simulink model "cruise_ground_up_final"  (R2021a)
settings: Solver=VariableStepAuto  StartTime=0  StopTime=10.0  RelTol=1e-3
model workspace (MAT data in the model file):
  aeroCoeff.Cl0 = 0
  aeroCoeff.Cl_beta = -0.036269164
  aeroCoeff.Cl_da = -0.1109919434
  aeroCoeff.Cl_dr = 0.1739783018
  aeroCoeff.Cl_p = -0.7949096926
  aeroCoeff.Cl_r = 0.2014971632
  aeroCoeff.Cm0 = 0
  aeroCoeff.Cm_alpha = -0.43
  aeroCoeff.Cm_de = -1.553
  aeroCoeff.Cm_q = -7.04
  aeroCoeff.Cn0 = 0
  aeroCoeff.Cn_beta = 0.048869199
  aeroCoeff.Cn_da = 0.0182026787
  aeroCoeff.Cn_dr = -0.3910440741
  aeroCoeff.Cn_p = -0.0359727396
  aeroCoeff.Cn_r = -0.0735610276
  aeroCoeff.Cx0 = 0
  aeroCoeff.Cx_alpha = 0.4653
  aeroCoeff.Cx_q = 0
  aeroCoeff.Cx_de = 0
  aeroCoeff.Cy0 = 0
  aeroCoeff.Cy_beta = -0.1609874369
  aeroCoeff.Cy_da = 0
  aeroCoeff.Cy_dr = 0.9151416544
  aeroCoeff.Cy_p = -0.0237997869
  aeroCoeff.Cy_r = 0.1375812867
  aeroCoeff.Cz0 = -1.136
  aeroCoeff.Cz_alpha = -5.16
  aeroCoeff.Cz_de = -0.6238
  aeroCoeff.Cz_q = -3.86
  aeroCoeff.Cx_u = -0.2199
  aeroCoeff.Cz_u = -2.272
  aeroCoeff.Cm_u = 0
  aeroCoeff.Cx_adot = 0
  aeroCoeff.Cz_adot = 1.43
  aeroCoeff.Cm_adot = -3.7
  aeroCoeff.V0 = 59.9
  environment.EarthRefAlt = 0
  initCond.x0 = [0 0 -1000]
  initCond.v0 = [59.9 0 0]
  initCond.euler0 = [0 0 0]
  initCond.w0 = [0 0 0]
  inputs0.time = 0
  inputs0.signals(1).dimensions = 1
  inputs0.signals(1).values = -0.104711430294
  inputs0.signals(2).dimensions = 1
  inputs0.signals(2).values = -0.0698725229544
  inputs0.signals(3).dimensions = 1
  inputs0.signals(3).values = -0.000215042330254
  states0.time = 0
  states0.signals(1).values = [0 0 -1000]
  states0.signals(1).dimensions = 3
  states0.signals(1).label = 'CSTATE'
  states0.signals(1).blockName = 'asb6DOFAirframeTemplate/6DOF EOM/6DOF (Euler Angles)/xe,ye,ze'
  states0.signals(1).stateName = ''
  states0.signals(1).inReferencedModel = 0
  states0.signals(1).sampleTime = [0 0]
  states0.signals(2).values = [0.128665353089 0.259337659946 -0.178947917154]
  states0.signals(2).dimensions = 3
  states0.signals(2).label = 'CSTATE'
  states0.signals(2).blockName = 'asb6DOFAirframeTemplate/6DOF EOM/6DOF (Euler Angles)/Calculate DCM &
    | Euler Angles/phi
    | theta
    | psi'
  states0.signals(2).stateName = ''
  states0.signals(2).inReferencedModel = 0
  states0.signals(2).sampleTime = [0 0]
  states0.signals(3).values = [36.9119692666 8.10720863264 8.82591882596]
  states0.signals(3).dimensions = 3
  states0.signals(3).label = 'CSTATE'
  states0.signals(3).blockName = 'asb6DOFAirframeTemplate/6DOF EOM/6DOF (Euler Angles)/ub,vb,wb'
  states0.signals(3).stateName = ''
  states0.signals(3).inReferencedModel = 0
  states0.signals(3).sampleTime = [0 0]
  states0.signals(4).values = [0 0 0]
  states0.signals(4).dimensions = 3
  states0.signals(4).label = 'CSTATE'
  states0.signals(4).blockName = 'asb6DOFAirframeTemplate/6DOF EOM/6DOF (Euler Angles)/p,q,r '
  states0.signals(4).stateName = ''
  states0.signals(4).inReferencedModel = 0
  states0.signals(4).sampleTime = [0 0]
  states0.signals(5).values = [0 0]
  states0.signals(5).dimensions = 2
  states0.signals(5).label = 'CSTATE'
  states0.signals(5).blockName = 'asb6DOFAirframeTemplate/Environment Model/Dryden Wind Turbulence Model 
    | (Continuous (+q +r))/Filters on velocities/Hwgw(s)/wg_p1'
  states0.signals(5).stateName = ''
  states0.signals(5).inReferencedModel = 0
  states0.signals(5).sampleTime = [0 0]
  states0.signals(6).values = [0 0]
  states0.signals(6).dimensions = 2
  states0.signals(6).label = 'CSTATE'
  states0.signals(6).blockName = 'asb6DOFAirframeTemplate/Environment Model/Dryden Wind Turbulence Model 
    | (Continuous (+q +r))/Filters on velocities/Hwgw(s)/wg_p2'
  states0.signals(6).stateName = ''
  states0.signals(6).inReferencedModel = 0
  states0.signals(6).sampleTime = [0 0]
  states0.signals(7).values = [0 0]
  states0.signals(7).dimensions = 2
  states0.signals(7).label = 'CSTATE'
  states0.signals(7).blockName = 'asb6DOFAirframeTemplate/Environment Model/Dryden Wind Turbulence Model 
    | (Continuous (+q +r))/Filters on velocities/Hvgw(s)/vg_p1'
  states0.signals(7).stateName = ''
  states0.signals(7).inReferencedModel = 0
  states0.signals(7).sampleTime = [0 0]
  states0.signals(8).values = [0 0]
  states0.signals(8).dimensions = 2
  states0.signals(8).label = 'CSTATE'
  states0.signals(8).blockName = 'asb6DOFAirframeTemplate/Environment Model/Dryden Wind Turbulence Model 
    | (Continuous (+q +r))/Filters on velocities/Hvgw(s)/vgw_p2'
  states0.signals(8).stateName = ''
  states0.signals(8).inReferencedModel = 0
  states0.signals(8).sampleTime = [0 0]
  states0.signals(9).values = [0 0]
  states0.signals(9).dimensions = 2
  states0.signals(9).label = 'CSTATE'
  states0.signals(9).blockName = 'asb6DOFAirframeTemplate/Environment Model/Dryden Wind Turbulence Model 
    | (Continuous (+q +r))/Filters on velocities/Hugw(s)/ug_p'
  states0.signals(9).stateName = ''
  states0.signals(9).inReferencedModel = 0
  states0.signals(9).sampleTime = [0 0]
  states0.signals(10).values = [0 0]
  states0.signals(10).dimensions = 2
  states0.signals(10).label = 'CSTATE'
  states0.signals(10).blockName = 'asb6DOFAirframeTemplate/Environment Model/Dryden Wind Turbulence Model 
    | (Continuous (+q +r))/Filters on angular rates/Hrgw/rgw_p'
  states0.signals(10).stateName = ''
  states0.signals(10).inReferencedModel = 0
  states0.signals(10).sampleTime = [0 0]
  states0.signals(11).values = [0 0]
  states0.signals(11).dimensions = 2
  states0.signals(11).label = 'CSTATE'
  states0.signals(11).blockName = 'asb6DOFAirframeTemplate/Environment Model/Dryden Wind Turbulence Model 
    | (Continuous (+q +r))/Filters on angular rates/Hqgw/qgw_p'
  states0.signals(11).stateName = ''
  states0.signals(11).inReferencedModel = 0
  states0.signals(11).sampleTime = [0 0]
  states0.signals(12).values = [0 0]
  states0.signals(12).dimensions = 2
  states0.signals(12).label = 'CSTATE'
  states0.signals(12).blockName = 'asb6DOFAirframeTemplate/Environment Model/Dryden Wind Turbulence Model 
    | (Continuous (+q +r))/Filters on angular rates/Hpgw/pgw_p'
  states0.signals(12).stateName = ''
  states0.signals(12).inReferencedModel = 0
  states0.signals(12).sampleTime = [0 0]
  vehicle.Sref = 24.2
  vehicle.cbar = 2.022
  vehicle.bref = 8.7036787674
  vehicle.CG = [0 0 0]
  vehicle.CP = [0 0 0]
  vehicle.inertia = [11509.7158987  0  121.163701749; 0  18221.7353845  0; -121.163701749  0  28644.1528969]
  vehicle.acMass = 4547.8
  vehicle.Thrust = 2300
  vehicle.aileron_max = 0.523598775598
  vehicle.aileron_min = -0.523598775598
  vehicle.elevator_max = 0.305432619099
  vehicle.elevator_min = -0.305432619099
  vehicle.rudder_max = 0.436332312999
  vehicle.rudder_min = -0.436332312999
values from neighbouring files (symbols this model uses):
  aeroCoeff = struct    [cruise_from_template_variables.m]    (also in cruise_ground_up_variables.m; cruise_ground_up_variables_cessna.m)
  vehicle = struct    [cruise_from_template_variables.m]    (also in cruise_ground_up_variables.m; cruise_ground_up_variables_cessna.m)
libraries: aerolibasang x2, pid_lib x2, aerolibadyn x1, aerolibatmos2 x1, shared6dof x1
settings Model: OrderedModelArguments=off  Creator=jakob  LastModifiedBy=jakob
settings DataIOCC: SaveFormat=StructureWithTime
settings OptimizationCC: BlockReduction=off  BufferReuse=off
settings DebuggingCC: AlgebraicLoopMsg=none  UnconnectedInputMsg=none  UnconnectedOutputMsg=none  UnconnectedLineMsg=none

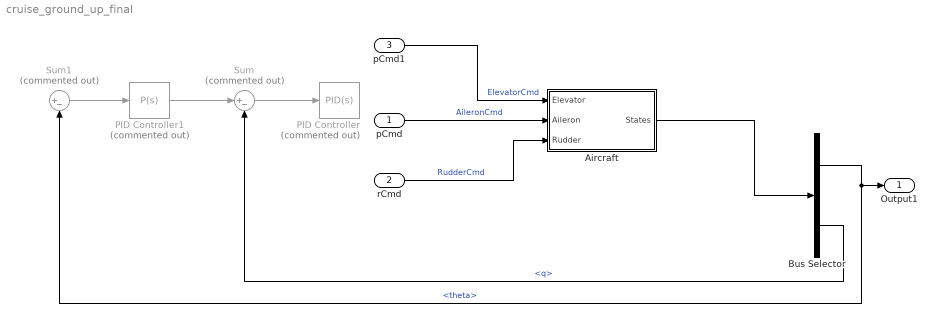
== system cruise_ground_up_final ==
  pCmd : Inport
  rCmd : Inport  Port=2
  pCmd1 : Inport  Port=3
  Aircraft : Subsystem
  Bus Selector : BusSelector  OutputSignals=phi,theta,psi,p,q,r
  PID Controller : pid_lib/PID Controller  Commented=on  Controller=PID  Form=Parallel  TimeDomain=Continuous-time  UseExternalTs=off  SampleTime=-1  IntegratorMethod=Forward Euler  FilterMethod=Forward Euler  ControllerParametersSource=internal  P=5.93921681747146  I=63.1505692304765  D=-0.00231186106807805  UseFilter=on  N=2569.01978214849  TunerSelectOption=Transfer Function Based (PID Tuner App)  InitialConditionSource=internal  InitialConditionForIntegrator=0  InitialConditionForFilter=0  DifferentiatorICPrevScaledInput=0  ExternalReset=none  TrackingMode=off  Kt=1  LimitOutput=off  SatLimitsSource=internal  UpperSaturationLimit=inf  LowerSaturationLimit=-inf  LinearizeAsGain=on  AntiWindupMode=none  Kb=1  POutMin=[]  POutMax=[]  IOutMin=[]  IOutMax=[]  DOutMin=[]  DOutMax=[]  NOutMin=[]  NOutMax=[]  SumOutMin=[]  SumOutMax=[]  SaturationOutMin=[]  SaturationOutMax=[]  PParamMin=[]  PParamMax=[]  IParamMin=[]  IParamMax=[]  DParamMin=[]  DParamMax=[]  NParamMin=[]  NParamMax=[]  KbParamMin=[]  KbParamMax=[]  KtParamMin=[]  KtParamMax=[]  KbOutMin=[]  KbOutMax=[]  KtOutMin=[]  KtOutMax=[]  IntegratorOutMin=[]  IntegratorOutMax=[]  FilterOutMin=[]  FilterOutMax=[]  SumI1OutMin=[]  SumI1OutMax=[]  SumI2OutMin=[]  SumI2OutMax=[]  SumI3OutMin=[]  SumI3OutMax=[]  SumI4OutMin=[]  SumI4OutMax=[]  SumDOutMin=[]  SumDOutMax=[]  DifferentiatorOutMin=[]  DifferentiatorOutMax=[]  FilterDiffOutCoefMin=[]  FilterDiffOutCoefMax=[]  ReciprocalOutMin=[]  ReciprocalOutMax=[]  SumDenOutMin=[]  SumDenOutMax=[]  SumNumOutMin=[]  SumNumOutMax=[]  DivideOutMin=[]  DivideOutMax=[]  UdiffTsProdOutMin=[]  UdiffTsProdOutMax=[]  NTsProdOutMin=[]  NTsProdOutMax=[]  UintegralTsProdOutMin=[]  UintegralTsProdOutMax=[]  UngainTsProdOutMin=[]  UngainTsProdOutMax=[]  IntegratorContinuousStateAttributes=''  IntegratorStateMustResolveToSignalObject=off  IntegratorRTWStateStorageClass=Auto  FilterContinuousStateAttributes=''  FilterStateMustResolveToSignalObject=off  FilterRTWStateStorageClass=Auto  ParallelPVariant=InternalParameters  IdealPVariant=Disabled  IVariant=InternalParameters  DVariant=InternalParameters  IntegratorVariant=Continuous  SatVariant=Disabled  AWVariant=Passthrough  PCopyVariant=Disabled  TRVariant=Disabled  FdbkBlocksVariant=Forward  IdealPFdbkVariant=Disabled  SatFdbkVariant=Disabled  DerivativeFilterVariant=ContFilter  NVariant=InternalParameters  NCopyVariant=Disabled  FilterICVariant=InternalICsFilter  IntegratorICVariant=InternalICs  ExternalResetVariant=Disabled  TRSumVariant=Passthrough  SumFdbkVariant=Disabled  SumVariant=Sum_PID  TsampFilterVariant=InternalTs  TsampNgainVariant=Passthrough  TsampIntegralVariant=Passthrough  ExternalSaturationOutDataTypeStr=Inherit: Same as second input
  PID Controller1 : pid_lib/PID Controller  Commented=on  Controller=P  Form=Parallel  TimeDomain=Continuous-time  UseExternalTs=off  SampleTime=-1  IntegratorMethod=Forward Euler  FilterMethod=Forward Euler  ControllerParametersSource=internal  P=3.47272160532588  I=1  D=0  UseFilter=on  N=100  TunerSelectOption=Transfer Function Based (PID Tuner App)  InitialConditionSource=internal  InitialConditionForIntegrator=0  InitialConditionForFilter=0  DifferentiatorICPrevScaledInput=0  ExternalReset=none  TrackingMode=off  Kt=1  LimitOutput=off  SatLimitsSource=internal  UpperSaturationLimit=inf  LowerSaturationLimit=-inf  LinearizeAsGain=on  AntiWindupMode=none  Kb=1  POutMin=[]  POutMax=[]  IOutMin=[]  IOutMax=[]  DOutMin=[]  DOutMax=[]  NOutMin=[]  NOutMax=[]  SumOutMin=[]  SumOutMax=[]  SaturationOutMin=[]  SaturationOutMax=[]  PParamMin=[]  PParamMax=[]  IParamMin=[]  IParamMax=[]  DParamMin=[]  DParamMax=[]  NParamMin=[]  NParamMax=[]  KbParamMin=[]  KbParamMax=[]  KtParamMin=[]  KtParamMax=[]  KbOutMin=[]  KbOutMax=[]  KtOutMin=[]  KtOutMax=[]  IntegratorOutMin=[]  IntegratorOutMax=[]  FilterOutMin=[]  FilterOutMax=[]  SumI1OutMin=[]  SumI1OutMax=[]  SumI2OutMin=[]  SumI2OutMax=[]  SumI3OutMin=[]  SumI3OutMax=[]  SumI4OutMin=[]  SumI4OutMax=[]  SumDOutMin=[]  SumDOutMax=[]  DifferentiatorOutMin=[]  DifferentiatorOutMax=[]  FilterDiffOutCoefMin=[]  FilterDiffOutCoefMax=[]  ReciprocalOutMin=[]  ReciprocalOutMax=[]  SumDenOutMin=[]  SumDenOutMax=[]  SumNumOutMin=[]  SumNumOutMax=[]  DivideOutMin=[]  DivideOutMax=[]  UdiffTsProdOutMin=[]  UdiffTsProdOutMax=[]  NTsProdOutMin=[]  NTsProdOutMax=[]  UintegralTsProdOutMin=[]  UintegralTsProdOutMax=[]  UngainTsProdOutMin=[]  UngainTsProdOutMax=[]  IntegratorContinuousStateAttributes=''  IntegratorStateMustResolveToSignalObject=off  IntegratorRTWStateStorageClass=Auto  FilterContinuousStateAttributes=''  FilterStateMustResolveToSignalObject=off  FilterRTWStateStorageClass=Auto  ParallelPVariant=InternalParameters  IdealPVariant=Disabled  IVariant=Disabled  DVariant=Disabled  IntegratorVariant=Disabled  SatVariant=Disabled  AWVariant=Disabled  PCopyVariant=Disabled  TRVariant=Disabled  FdbkBlocksVariant=Forward  IdealPFdbkVariant=Disabled  SatFdbkVariant=Disabled  DerivativeFilterVariant=Disabled  NVariant=Disabled  NCopyVariant=Disabled_SignalSpec  FilterICVariant=Disabled  IntegratorICVariant=Disabled  ExternalResetVariant=Disabled  TRSumVariant=Passthrough  SumFdbkVariant=Disabled  SumVariant=Passthrough_P  TsampFilterVariant=InternalTs  TsampNgainVariant=Passthrough  TsampIntegralVariant=Disabled_SignalSpec  ExternalSaturationOutDataTypeStr=Inherit: Same as second input
  Sum : Sum  Commented=on  Inputs=|+-
  Sum1 : Sum  Commented=on  Inputs=|+-
  Output1 : Outport
  wires:
  Aircraft/1(States) -> Bus Selector/1
  pCmd/1 -> Aircraft/2(Aileron)  "AileronCmd"
  rCmd/1 -> Aircraft/3(Rudder)  "RudderCmd"
  Sum/1 -> PID Controller/1
  Bus Selector/5 -> Sum/2  "<q>"
  Sum1/1 -> PID Controller1/1
  PID Controller1/1 -> Sum/1
  Bus Selector/2 -> Output1/1, Sum1/2  "<theta>"
  pCmd1/1 -> Aircraft/1(Elevator)  "ElevatorCmd"

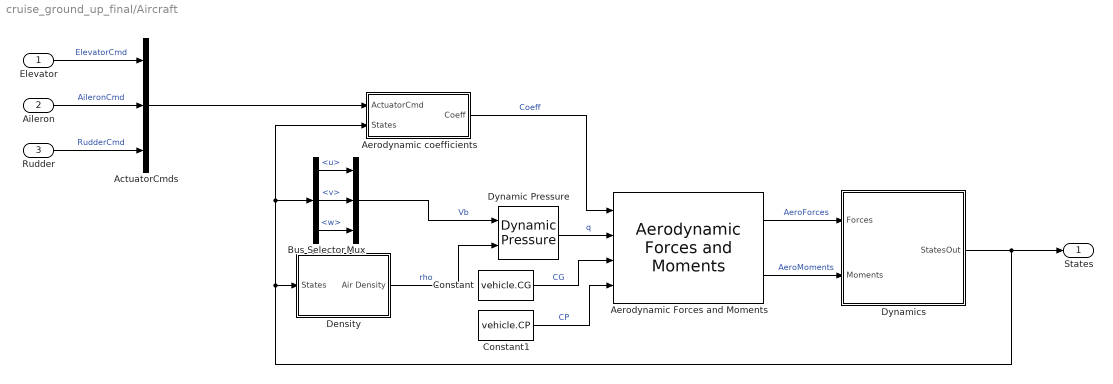
== system cruise_ground_up_final/Aircraft ==
  Elevator : Inport
  Aileron : Inport  Port=2
  Rudder : Inport  Port=3
  ActuatorCmds : BusCreator  Inputs=3
  "Aerodynamic Forces and Moments " : aerolibadyn/Aerodynamic Forces and Moments   inputAxes=Body  outputForceAxes=Body  outputMomentAxes=Body  S=vehicle.Sref  b=vehicle.bref  cbar=vehicle.cbar
  Aerodynamic coefficients : Subsystem
  Bus Selector : BusSelector  OutputSignals=u,v,w
  Constant : Constant  Value=vehicle.CG
  Constant1 : Constant  Value=vehicle.CP
  Density : Subsystem
  Dynamic Pressure : aerolibasang/Dynamic Pressure
  Dynamics : Subsystem
  Mux : Mux  Inputs=3
  States : Outport
  wires:
  "Aerodynamic Forces and Moments "/1 -> Dynamics/1(Forces)  "AeroForces"
  Aileron/1 -> ActuatorCmds/2  "AileronCmd"
  ActuatorCmds/1 -> Aerodynamic coefficients/1(ActuatorCmd)
  Rudder/1 -> ActuatorCmds/3  "RudderCmd"
  Dynamic Pressure/1 -> "Aerodynamic Forces and Moments "/2  "q"
  Elevator/1 -> ActuatorCmds/1  "ElevatorCmd"
  Aerodynamic coefficients/1(Coeff) -> "Aerodynamic Forces and Moments "/1  "Coeff"
  Dynamics/1(StatesOut) -> States/1, Aerodynamic coefficients/2(States), Bus Selector/1, Density/1(States)
  "Aerodynamic Forces and Moments "/2 -> Dynamics/2(Moments)  "AeroMoments"
  Density/1(Air Density) -> Dynamic Pressure/2  "rho"
  Constant/1 -> "Aerodynamic Forces and Moments "/3  "CG"
  Mux/1 -> Dynamic Pressure/1  "Vb"
  Constant1/1 -> "Aerodynamic Forces and Moments "/4  "CP"
  Bus Selector/2 -> Mux/2  "<v>"
  Bus Selector/1 -> Mux/1  "<u>"
  Bus Selector/3 -> Mux/3  "<w>"

== system cruise_ground_up_final/Aircraft/Aerodynamic coefficients ==
  ActuatorCmd : Inport
  States : Inport  Port=2
  Control derivatives : Subsystem
  Stability derivatives : Subsystem
  Sum : Sum  Inputs=|++
  Coeff : Outport
  wires:
  Sum/1 -> Coeff/1
  Stability derivatives/1(Coeff) -> Sum/2
  Control derivatives/1(Coeff) -> Sum/1
  States/1 -> Stability derivatives/1(StatesOut)
  ActuatorCmd/1 -> Control derivatives/1(ActuatorCmd)

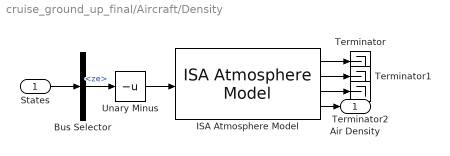
== system cruise_ground_up_final/Aircraft/Density ==
  States : Inport
  Bus Selector : BusSelector  OutputSignals=ze
  ISA Atmosphere Model : aerolibatmos2/ISA Atmosphere Model  custom=off  g=9.80665  gamma=1.4  R=287.0531  L=0.0065  h_trop=11000  h_strat=20000  rho0=1.225  P0=101325  T0=288.15  h0=0
  Terminator : Terminator
  Terminator1 : Terminator
  Terminator2 : Terminator
  Unary Minus : UnaryMinus
  Air Density : Outport
  wires:
  ISA Atmosphere Model/3 -> Terminator2/1
  ISA Atmosphere Model/2 -> Terminator1/1
  ISA Atmosphere Model/4 -> Air Density/1
  Bus Selector/1 -> Unary Minus/1  "<ze>"
  Unary Minus/1 -> ISA Atmosphere Model/1
  ISA Atmosphere Model/1 -> Terminator/1
  States/1 -> Bus Selector/1

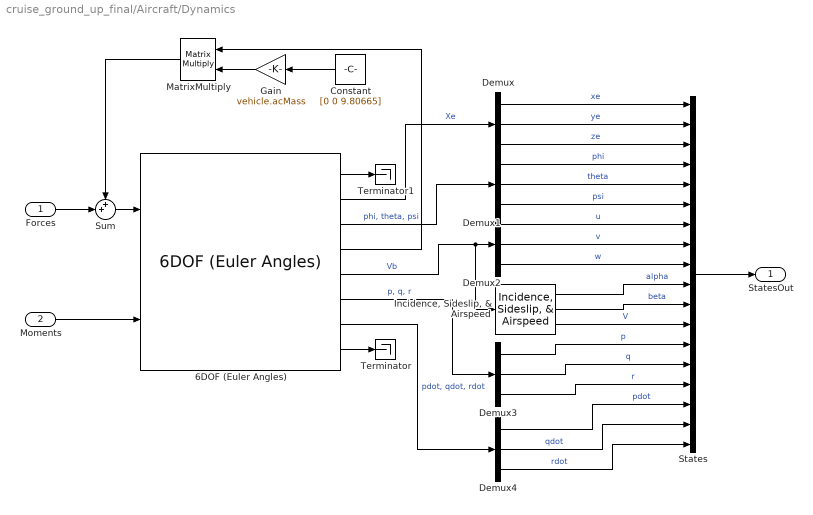
== system cruise_ground_up_final/Aircraft/Dynamics ==
  Forces : Inport
  Moments : Inport  Port=2
  6DOF (Euler Angles) : shared6dof/6DOF (Euler Angles)  units=Metric (MKS)  mtype=Fixed  rep=Euler Angles  xme_0=initCond.x0  Vm_0=initCond.v0  eul_0=initCond.euler0  pm_0=initCond.w0  mass_0=vehicle.acMass  mass_e=0.5  mass_f=2.0  inertia=vehicle.inertia  inertia_e=eye(3)  inertia_f=2*eye(3)  k_quat=1.0  vre_flag=on  abi_flag=off  aMode=0  xme_statename=''  Vm_statename=''  eul_statename=''  quat_statename=''  pm_statename=''  mass_statename=''
      settings: SourceProductBaseCode=AE,PW,DR,MT,UV,VE
  Constant : Constant  Value=[0 0 9.80665]
  Demux{,1..4} (5 alike) : Demux  Outputs=3
  Gain : Gain  Gain=vehicle.acMass
  "Incidence, Sideslip, & Airspeed" : aerolibasang/Incidence, Sideslip, & Airspeed
  MatrixMultiply : Product  Multiplication=Matrix(*)
  States : BusCreator  Inputs=18
  Sum : Sum  Inputs=++|
  Terminator : Terminator
  Terminator1 : Terminator
  StatesOut : Outport
  wires:
  Demux1/1 -> States/4  "phi"
  Demux1/3 -> States/6  "psi"
  6DOF (Euler Angles)/7 -> Demux4/1  "pdot, qdot, rdot"
  Demux2/2 -> States/8  "v"
  Demux/3 -> States/3  "ze"
  Demux3/2 -> States/14  "q"
  Demux3/3 -> States/15  "r"
  6DOF (Euler Angles)/8 -> Terminator/1
  6DOF (Euler Angles)/5 -> "Incidence, Sideslip, & Airspeed"/1, Demux2/1  "Vb"
  6DOF (Euler Angles)/3 -> Demux1/1  "phi, theta, psi"
  Demux/2 -> States/2  "ye"
  Demux2/1 -> States/7  "u"
  Demux4/3 -> States/18  "rdot"
  Demux1/2 -> States/5  "theta"
  Demux4/2 -> States/17  "qdot"
  Demux4/1 -> States/16  "pdot"
  6DOF (Euler Angles)/2 -> Demux/1  "Xe"
  Constant/1 -> Gain/1
  6DOF (Euler Angles)/6 -> Demux3/1  "p, q, r"
  States/1 -> StatesOut/1
  Demux3/1 -> States/13  "p"
  Demux2/3 -> States/9  "w"
  Demux/1 -> States/1  "xe"
  6DOF (Euler Angles)/1 -> Terminator1/1
  Moments/1 -> 6DOF (Euler Angles)/2
  Sum/1 -> 6DOF (Euler Angles)/1
  Forces/1 -> Sum/2
  MatrixMultiply/1 -> Sum/1
  "Incidence, Sideslip, & Airspeed"/1 -> States/10  "alpha"
  "Incidence, Sideslip, & Airspeed"/2 -> States/11  "beta"
  "Incidence, Sideslip, & Airspeed"/3 -> States/12  "V"
  Gain/1 -> MatrixMultiply/2
  6DOF (Euler Angles)/4 -> MatrixMultiply/1

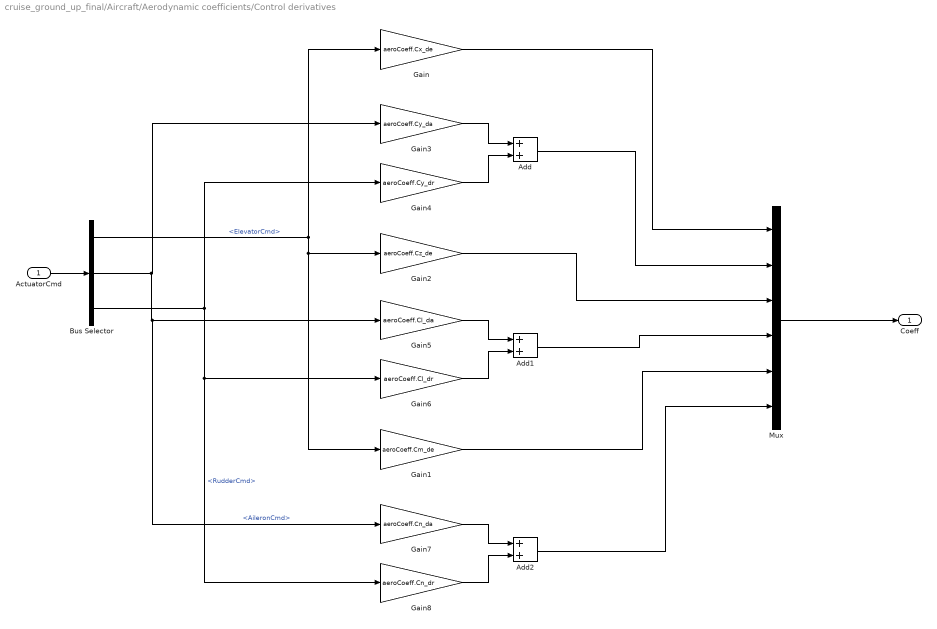
== system cruise_ground_up_final/Aircraft/Aerodynamic coefficients/Control derivatives ==
  ActuatorCmd : Inport
  Add : Sum
  Add1 : Sum
  Add2 : Sum
  Bus Selector : BusSelector  OutputSignals=ElevatorCmd,AileronCmd,RudderCmd
  Gain : Gain  Gain=aeroCoeff.Cx_de
  Gain1 : Gain  Gain=aeroCoeff.Cm_de
  Gain2 : Gain  Gain=aeroCoeff.Cz_de
  Gain3 : Gain  Gain=aeroCoeff.Cy_da
  Gain4 : Gain  Gain=aeroCoeff.Cy_dr
  Gain5 : Gain  Gain=aeroCoeff.Cl_da
  Gain6 : Gain  Gain=aeroCoeff.Cl_dr
  Gain7 : Gain  Gain=aeroCoeff.Cn_da
  Gain8 : Gain  Gain=aeroCoeff.Cn_dr
  Mux : Mux  Inputs=6
  Coeff : Outport
  wires:
  ActuatorCmd/1 -> Bus Selector/1
  Bus Selector/1 -> Gain/1, Gain1/1, Gain2/1  "<ElevatorCmd>"
  Gain/1 -> Mux/1
  Gain2/1 -> Mux/3
  Gain1/1 -> Mux/5
  Gain3/1 -> Add/1
  Gain4/1 -> Add/2
  Bus Selector/2 -> Gain7/1, Gain5/1, Gain3/1  "<AileronCmd>"
  Add/1 -> Mux/2
  Bus Selector/3 -> Gain8/1, Gain6/1, Gain4/1  "<RudderCmd>"
  Gain5/1 -> Add1/1
  Gain6/1 -> Add1/2
  Add1/1 -> Mux/4
  Gain7/1 -> Add2/1
  Gain8/1 -> Add2/2
  Add2/1 -> Mux/6
  Mux/1 -> Coeff/1

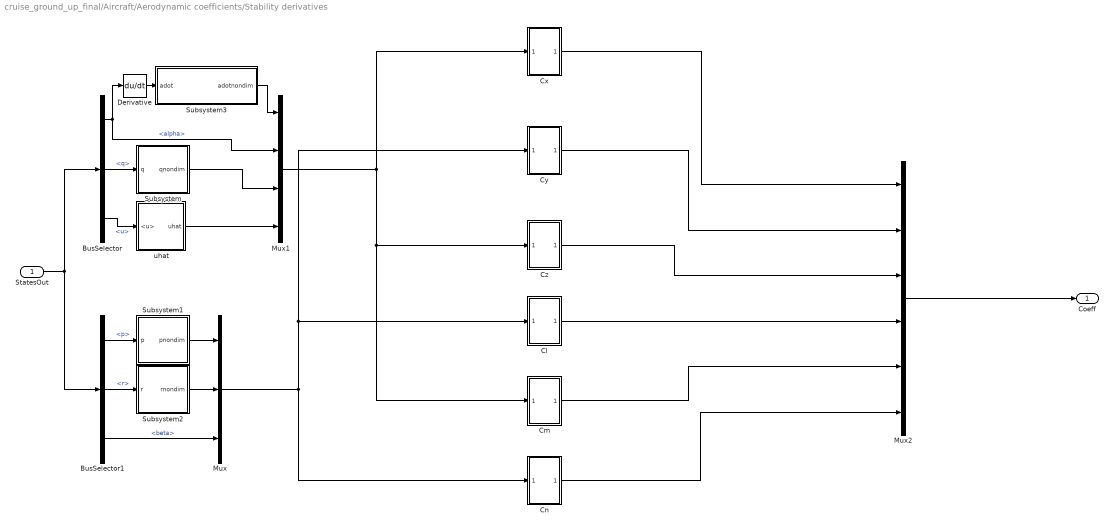
== system cruise_ground_up_final/Aircraft/Aerodynamic coefficients/Stability derivatives ==
  StatesOut : Inport
  BusSelector : BusSelector  OutputSignals=alpha,q,u
  BusSelector1 : BusSelector  OutputSignals=p,r,beta
  Cl : Subsystem
  Cm : Subsystem
  Cn : Subsystem
  Cx : Subsystem
  Cy : Subsystem
  Cz : Subsystem
  Derivative : Derivative
  Mux : Mux  Inputs=3
  Mux1 : Mux
  Mux2 : Mux  Inputs=6
  Subsystem : Subsystem
  Subsystem1 : Subsystem
  Subsystem2 : Subsystem
  Subsystem3 : Subsystem
  uhat : Subsystem
  Coeff : Outport
  wires:
  StatesOut/1 -> BusSelector1/1, BusSelector/1
  BusSelector/3 -> uhat/1(<u>)  "<u>"
  BusSelector1/3 -> Mux/3  "<beta>"
  uhat/1(uhat) -> Mux1/4
  BusSelector/1 -> Derivative/1, Mux1/2  "<alpha>"
  BusSelector/2 -> Subsystem/1(q)  "<q>"
  Subsystem/1(qnondim) -> Mux1/3
  BusSelector1/1 -> Subsystem1/1(p)  "<p>"
  Subsystem1/1(pnondim) -> Mux/1
  BusSelector1/2 -> Subsystem2/1(r)  "<r>"
  Subsystem2/1(rnondim) -> Mux/2
  Mux1/1 -> Cx/1(In1), Cm/1(In1), Cz/1(In1)
  Mux/1 -> Cn/1(In1), Cl/1(In1), Cy/1(In1)
  Mux2/1 -> Coeff/1
  Cx/1(Out1) -> Mux2/1
  Cy/1(Out1) -> Mux2/2
  Cz/1(Out1) -> Mux2/3
  Cl/1(Out1) -> Mux2/4
  Cm/1(Out1) -> Mux2/5
  Cn/1(Out1) -> Mux2/6
  Derivative/1 -> Subsystem3/1(adot)
  Subsystem3/1(adotnondim) -> Mux1/1

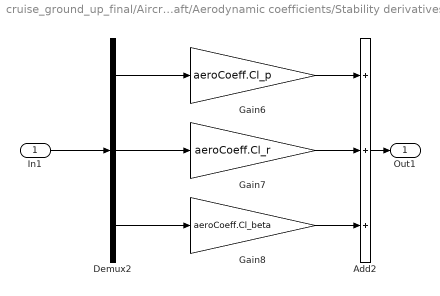
== system cruise_ground_up_final/Aircraft/Aerodynamic coefficients/Stability derivatives/Cl ==
  In1 : Inport
  Add2 : Sum  Inputs=+++
  Demux2 : Demux  Outputs=3
  Gain6 : Gain  Gain=aeroCoeff.Cl_p
  Gain7 : Gain  Gain=aeroCoeff.Cl_r
  Gain8 : Gain  Gain=aeroCoeff.Cl_beta
  Out1 : Outport
  wires:
  Demux2/2 -> Gain7/1
  Gain6/1 -> Add2/1
  In1/1 -> Demux2/1
  Add2/1 -> Out1/1
  Gain8/1 -> Add2/3
  Demux2/3 -> Gain8/1
  Demux2/1 -> Gain6/1
  Gain7/1 -> Add2/2

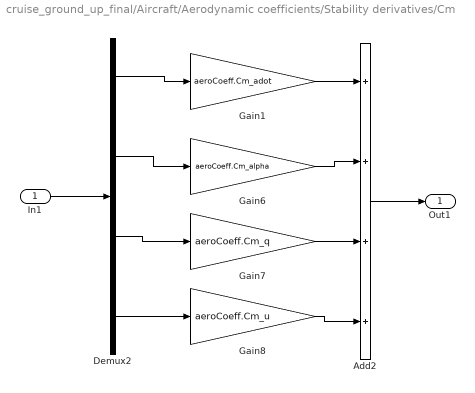
== system cruise_ground_up_final/Aircraft/Aerodynamic coefficients/Stability derivatives/Cm ==
  In1 : Inport
  Add2 : Sum  Inputs=++++
  Demux2 : Demux
  Gain1 : Gain  Gain=aeroCoeff.Cm_adot
  Gain6 : Gain  Gain=aeroCoeff.Cm_alpha
  Gain7 : Gain  Gain=aeroCoeff.Cm_q
  Gain8 : Gain  Gain=aeroCoeff.Cm_u
  Out1 : Outport
  wires:
  Demux2/3 -> Gain7/1
  Gain6/1 -> Add2/2
  In1/1 -> Demux2/1
  Add2/1 -> Out1/1
  Gain8/1 -> Add2/4
  Demux2/4 -> Gain8/1
  Demux2/2 -> Gain6/1
  Gain7/1 -> Add2/3
  Demux2/1 -> Gain1/1
  Gain1/1 -> Add2/1

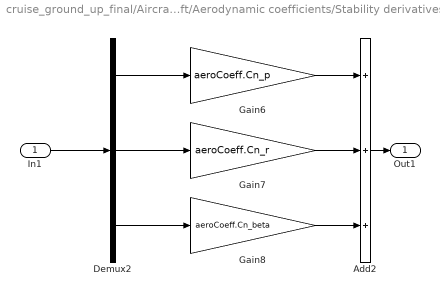
== system cruise_ground_up_final/Aircraft/Aerodynamic coefficients/Stability derivatives/Cn ==
  In1 : Inport
  Add2 : Sum  Inputs=+++
  Demux2 : Demux  Outputs=3
  Gain6 : Gain  Gain=aeroCoeff.Cn_p
  Gain7 : Gain  Gain=aeroCoeff.Cn_r
  Gain8 : Gain  Gain=aeroCoeff.Cn_beta
  Out1 : Outport
  wires:
  Demux2/2 -> Gain7/1
  Gain6/1 -> Add2/1
  In1/1 -> Demux2/1
  Add2/1 -> Out1/1
  Gain8/1 -> Add2/3
  Demux2/3 -> Gain8/1
  Demux2/1 -> Gain6/1
  Gain7/1 -> Add2/2

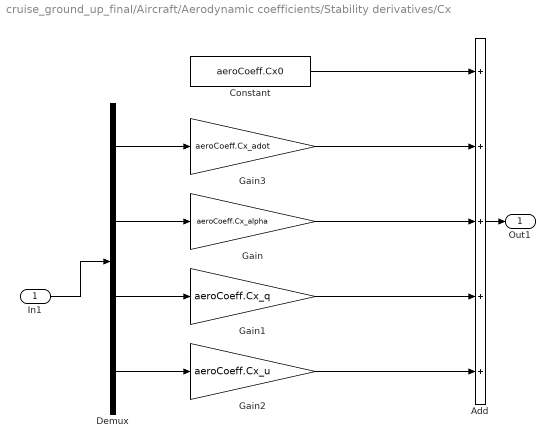
== system cruise_ground_up_final/Aircraft/Aerodynamic coefficients/Stability derivatives/Cx ==
  In1 : Inport
  Add : Sum  Inputs=+++++
  Constant : Constant  Value=aeroCoeff.Cx0
  Demux : Demux
  Gain : Gain  Gain=aeroCoeff.Cx_alpha
  Gain1 : Gain  Gain=aeroCoeff.Cx_q
  Gain2 : Gain  Gain=aeroCoeff.Cx_u
  Gain3 : Gain  Gain=aeroCoeff.Cx_adot
  Out1 : Outport
  wires:
  Gain/1 -> Add/3
  Gain2/1 -> Add/5
  Add/1 -> Out1/1
  Demux/4 -> Gain2/1
  Demux/3 -> Gain1/1
  Gain1/1 -> Add/4
  In1/1 -> Demux/1
  Constant/1 -> Add/1
  Demux/2 -> Gain/1
  Gain3/1 -> Add/2
  Demux/1 -> Gain3/1

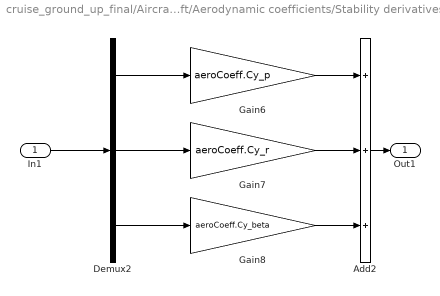
== system cruise_ground_up_final/Aircraft/Aerodynamic coefficients/Stability derivatives/Cy ==
  In1 : Inport
  Add2 : Sum  Inputs=+++
  Demux2 : Demux  Outputs=3
  Gain6 : Gain  Gain=aeroCoeff.Cy_p
  Gain7 : Gain  Gain=aeroCoeff.Cy_r
  Gain8 : Gain  Gain=aeroCoeff.Cy_beta
  Out1 : Outport
  wires:
  Demux2/2 -> Gain7/1
  Gain6/1 -> Add2/1
  In1/1 -> Demux2/1
  Add2/1 -> Out1/1
  Gain8/1 -> Add2/3
  Demux2/3 -> Gain8/1
  Demux2/1 -> Gain6/1
  Gain7/1 -> Add2/2

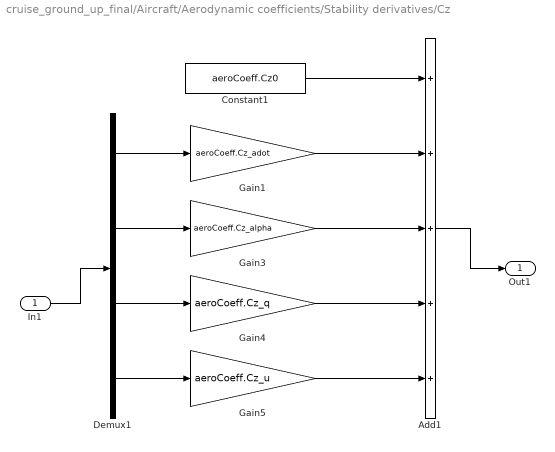
== system cruise_ground_up_final/Aircraft/Aerodynamic coefficients/Stability derivatives/Cz ==
  In1 : Inport
  Add1 : Sum  Inputs=+++++
  Constant1 : Constant  Value=aeroCoeff.Cz0
  Demux1 : Demux
  Gain1 : Gain  Gain=aeroCoeff.Cz_adot
  Gain3 : Gain  Gain=aeroCoeff.Cz_alpha
  Gain4 : Gain  Gain=aeroCoeff.Cz_q
  Gain5 : Gain  Gain=aeroCoeff.Cz_u
  Out1 : Outport
  wires:
  Demux1/3 -> Gain4/1
  Demux1/2 -> Gain3/1
  Gain5/1 -> Add1/5
  Gain4/1 -> Add1/4
  Constant1/1 -> Add1/1
  In1/1 -> Demux1/1
  Demux1/4 -> Gain5/1
  Gain3/1 -> Add1/3
  Add1/1 -> Out1/1
  Demux1/1 -> Gain1/1
  Gain1/1 -> Add1/2

== system cruise_ground_up_final/Aircraft/Aerodynamic coefficients/Stability derivatives/Subsystem ==
  q : Inport
  Constant : Constant  Value=aeroCoeff.V0
  Constant1 : Constant  Value=vehicle.cbar
  Divide : Product  Inputs=*/
  Product : Product
  qnondim : Outport
  wires:
  Product/1 -> Divide/1
  Divide/1 -> qnondim/1
  Constant1/1 -> Product/1
  q/1 -> Product/2
  Constant/1 -> Divide/2

== system cruise_ground_up_final/Aircraft/Aerodynamic coefficients/Stability derivatives/Subsystem1 ==
  p : Inport
  Constant : Constant  Value=aeroCoeff.V0
  Constant1 : Constant  Value=vehicle.bref
  Divide : Product  Inputs=*/
  Gain : Gain  Gain=2
  Product : Product
  pnondim : Outport
  wires:
  Product/1 -> Divide/1
  Divide/1 -> pnondim/1
  Constant1/1 -> Product/1
  p/1 -> Product/2
  Gain/1 -> Divide/2
  Constant/1 -> Gain/1

== system cruise_ground_up_final/Aircraft/Aerodynamic coefficients/Stability derivatives/Subsystem2 ==
  r : Inport
  Constant : Constant  Value=aeroCoeff.V0
  Constant1 : Constant  Value=vehicle.bref
  Divide : Product  Inputs=*/
  Gain : Gain  Gain=2
  Product : Product
  rnondim : Outport
  wires:
  Product/1 -> Divide/1
  Divide/1 -> rnondim/1
  Constant1/1 -> Product/1
  Gain/1 -> Divide/2
  r/1 -> Product/2
  Constant/1 -> Gain/1

== system cruise_ground_up_final/Aircraft/Aerodynamic coefficients/Stability derivatives/Subsystem3 ==
  adot : Inport
  Constant : Constant  Value=aeroCoeff.V0
  Constant1 : Constant  Value=vehicle.cbar
  Divide : Product  Inputs=*/
  Product : Product
  adotnondim : Outport
  wires:
  Product/1 -> Divide/1
  Divide/1 -> adotnondim/1
  Constant1/1 -> Product/1
  adot/1 -> Product/2
  Constant/1 -> Divide/2

== system cruise_ground_up_final/Aircraft/Aerodynamic coefficients/Stability derivatives/uhat ==
  <u> : Inport
  Constant : Constant  Value=aeroCoeff.V0
  Divide : Product  Inputs=*/
  Subtract : Sum  Inputs=+-
  uhat : Outport
  wires:
  Constant/1 -> Divide/2, Subtract/2
  Subtract/1 -> Divide/1
  <u>/1 -> Subtract/1
  Divide/1 -> uhat/1
